simulink model "NGGenset_Test_System"  (R2013a)
settings: Solver=ode3  SolverMode=SingleTasking  StartTime=0.0  StopTime=150  FixedStep=Ts  RelTol=1e-3
PostLoadFcn:
  | Ts=50e-6;SIM_HIL=0;
InitFcn:
  | Ts=50e-6;SIM_HIL=0;
model workspace (MAT data in the model file):
  handle : class17 (value not decoded)
undefined symbols (not defined in the file): DiscIntNeverNeededParam, fdesignblkfcn, gcbh, Gen_900kW_external_control, Generator, HIL_GenSet, Left, NG_Genset_lib, ph, type, V
libraries: powerlib x33, simulink x30, powerlib_extras x24, rtio_opalrt_common x21, simulink_extras x6, dspsigops x6, breakers_1ph_3ph x6, rtio_generic_modbus x6, cables_lib x5, rteventslib x4, rtlab x2, ssn_lib x2
(part 3 of 4)

== system NGGenset_Test_System/SC_Console/Woodward/16TSDIn//16 TSDOut GR3/Din//Dout ch24-31 ==
  Bus Creator4 : BusCreator  Inputs=8
  times25 : Constant  Value=[0.05 0.15 0.25 0.35]
  times26 : Constant  Value=[0.1 0.2 0.3 0.4]
  times27 : Constant  Value=[0.15 0.25 0.35 0.45]
  times28 : Constant  Value=[0.2 0.3 0.4 0.5]
  times29 : Constant  Value=[0.25 0.35 0.45 0.55]
  times30 : Constant  Value=[0.3 0.4 0.5 0.6]
  times31 : Constant  Value=[0.3 0.4 0.5 0.6]
  times32 : Constant  Value=[0 0.1 0.2 0.3]
  Out1 : Outport
  wires:
  Bus Creator4/1 -> Out1/1
  times31/1 -> Bus Creator4/8  "times32"
  times30/1 -> Bus Creator4/7  "times31"
  times29/1 -> Bus Creator4/6  "times30"
  times28/1 -> Bus Creator4/5  "times29"
  times27/1 -> Bus Creator4/4  "times28"
  times26/1 -> Bus Creator4/3  "times27"
  times25/1 -> Bus Creator4/2  "times26"
  times32/1 -> Bus Creator4/1  "times25"

== system NGGenset_Test_System/SC_Console/Woodward/16TSDIn//16 TSDOut GR3/Dout state ctrl ==
  Bus Creator : BusCreator  Inputs=2
  Dout_CH16_CH23 : Subsystem
  Dout_CH24_CH31 : Subsystem
  Event State OUT : Outport
  wires:
  Dout_CH24_CH31/1(Dout_CH8_CH15) -> Bus Creator/2  "CH24-31"
  Dout_CH16_CH23/1(Dout_CH8_CH15) -> Bus Creator/1  "CH16-23"
  Bus Creator/1 -> Event State OUT/1

== system NGGenset_Test_System/SM_Master/Generator/NG Genset 3.5MVA/3.5MVA Generator with Primary Controllers1 ==
  wref : Inport
  Vtref : Inport  Port=2
  Enable : Inport  Port=3
  w_meas_Woodward : Inport  Port=4
  V_meas_Woodward : Inport  Port=5
  Woodward_Enable : Inport  Port=6
  Bus Creator1 : BusCreator
  Bus Creator3 : BusCreator  Inputs=3
  Bus Selector : BusSelector  OutputSignals=Vf_before,Vf_after
  NG Engine Speed & Voltage Control fast : Subsystem
  Synchronous Machine pu Fundamental : powerlib/Machines/Synchronous Machine pu Fundamental  PresetModel=No  MechanicalLoad=Mechanical power Pm  ShowDetailedParameters=on  RotorType=Salient-pole  NominalParameters=[3.5e+006 13800 60]  Stator=[0.008979 0.05 2.35 1.72]  Field=[0.00206 0.511]  Dampers2=[0.0652, 0.5134, 0.0287, 0.2553, 7.765e-3, 0.9167 ]  Dampers1=[0.2826 3.738 0.02545 0.2392]  Mechanical=[0.3468 0.009238 2]  PolePairs=2  InitialConditions="[ -99  0  0  0  0  0  0  0  0 ]"  SetSaturation=off  Saturation=[0.6404,0.7127,0.8441,0.9214,0.9956,1.082,1.19,1.316,1.457;0.7,0.7698,0.8872,0.9466,0.9969,1.046,1.1,1.151,1.201]  Units=per unit fundamental parameters  LoadFlowParameters=[1,0,0,0,0]  TsPowergui=0  TsBlock=-1  IterativeModel=Forward Euler  BusType=swing  Pref=0  Qref=0  Qmin=-inf  Qmax=inf  PLF=0  QLF=0
  A : PMIOPort  Port=1  Side=Right
  B : PMIOPort  Port=2  Side=Right
  C : PMIOPort  Port=3  Side=Right
  m : Outport
  Primary : Outport  Port=2
  Thermal data : Outport  Port=3
  wires:
  Woodward_Enable/1 -> NG Engine Speed & Voltage Control fast/7(Woodward Enable)
  Bus Creator3/1 -> Bus Creator1/2  "Vf"
  Bus Selector/2 -> Bus Creator3/3  "<Vf_after>"
  Bus Selector/1 -> Bus Creator3/2  "<Vf_before>"
  NG Engine Speed & Voltage Control fast/5(Misc) -> Bus Selector/1
  Bus Creator1/1 -> Primary/1
  NG Engine Speed & Voltage Control fast/4(w) -> Bus Creator1/4  "w"
  NG Engine Speed & Voltage Control fast/3(Vt) -> Bus Creator1/3  "vt"
  V_meas_Woodward/1 -> NG Engine Speed & Voltage Control fast/6(V_meas_Wood)
  w_meas_Woodward/1 -> NG Engine Speed & Voltage Control fast/5(w_meas_Wood)
  Synchronous Machine pu Fundamental/1 -> m/1, NG Engine Speed & Voltage Control fast/4(m)
  Enable/1 -> NG Engine Speed & Voltage Control fast/3(Generator Enable)
  NG Engine Speed & Voltage Control fast/1(Pm) -> Bus Creator1/1, Synchronous Machine pu Fundamental/1  "Pm"
  NG Engine Speed & Voltage Control fast/2(Vf) -> Bus Creator3/1, Synchronous Machine pu Fundamental/2  "vf"
  wref/1 -> NG Engine Speed & Voltage Control fast/1(wref)
  Vtref/1 -> NG Engine Speed & Voltage Control fast/2(Vtref)
  NG Engine Speed & Voltage Control fast/6(Themal data) -> Thermal data/1
  connections:
  Synchronous Machine pu Fundamental/RConn1 -- A/RConn1
  Synchronous Machine pu Fundamental/RConn2 -- B/RConn1
  Synchronous Machine pu Fundamental/RConn3 -- C/RConn1

== system NGGenset_Test_System/SM_Master/Generator/NG Genset 3.5MVA/Interface between Woodward Controller and simated generator ==
  note: Note: This may need a different scaling because it is the reference signal.
      | Reference has to be between 0.95 and 1.05 pu in order to be in tolerance.
  Woodward for wref : Inport
  Woodward for Vref : Inport  Port=2
  Add2 : Sum
  Add3 : Sum
  Gain2 : Gain
  Gain3 : Gain
  Mux1 : Mux  Inputs=2
  Vref_set : Constant  Value=0
  wref_set : Constant  Value=0
  wref,Vref : Outport
  wires:
  Gain2/1 -> Add2/1  "bias"
  Add2/1 -> Mux1/1
  Gain3/1 -> Add3/1  "bias"
  Vref_set/1 -> Add3/2
  Add3/1 -> Mux1/2
  Woodward for wref/1 -> Gain2/1
  Mux1/1 -> wref,Vref/1  "hardware"
  Woodward for Vref/1 -> Gain3/1
  wref_set/1 -> Add2/2

== system NGGenset_Test_System/SM_Master/Generator/NG Genset 3.5MVA/Simulated Generator Controller 3.5 MW ==
  Pref : Inport
  Qref : Inport  Port=2
  mode : Inport  Port=3
  set_vtref : Inport  Port=4
  set_wref : Inport  Port=5
  gen_m : Inport  Port=6
  Bus Selector1 : BusSelector  OutputSignals="Output active power   Peo (pu),Output reactive power  Qeo (pu)"
  Multiport Switch1 : MultiPortSwitch  DiagnosticForDefault=Warning
  Mux1 : Mux  Inputs=2
  Mux2 : Mux  Inputs=2
  Mux3 : Mux  Inputs=2
  PQ control : Subsystem
  PV control : Subsystem
  "wref, Vref" : Outport
  wires:
  Bus Selector1/1 -> PQ control/2(P (pu)), PV control/2(P (pu))  "<Output active power   Peo (pu)>"
  gen_m/1 -> Bus Selector1/1
  PQ control/1(w_ref (pu)) -> Mux1/1
  PQ control/2(V_ref (pu)) -> Mux1/2
  PV control/1(w_ref (pu)) -> Mux2/1
  set_vtref/1 -> Mux2/2, Mux3/2
  Mux1/1 -> Multiport Switch1/2
  Mux2/1 -> Multiport Switch1/3
  Mux3/1 -> Multiport Switch1/4
  Pref/1 -> PQ control/1(P_ref (pu)), PV control/1(P_ref (pu))
  Bus Selector1/2 -> PQ control/4(Q (pu))  "<Output reactive power  Qeo (pu)>"
  set_wref/1 -> Mux3/1
  Qref/1 -> PQ control/3(Q_ref (pu))
  mode/1 -> Multiport Switch1/1
  Multiport Switch1/1 -> "wref, Vref"/1

== system NGGenset_Test_System/SM_Master/Generator/NG Genset 3.5MVA/StabilityL ==
  Constant Load : powerlib/Elements/Three-Phase Parallel RLC Load  LConnTagsString=A|B|C  Configuration=Y (grounded)  NominalVoltage=v  NominalFrequency=60  ActivePower=kVA*1E3*pf  InductivePower=kVA*1E3*sqrt(1-pf^2)  CapacitivePower=0  Measurements=None  LoadType=constant Z
  A : PMIOPort  Port=1  Side=Left
  B : PMIOPort  Port=2  Side=Left
  C : PMIOPort  Port=3  Side=Left
  connections:
  A/RConn1 -- Constant Load/LConn1
  B/RConn1 -- Constant Load/LConn2
  C/RConn1 -- Constant Load/LConn3

== system NGGenset_Test_System/SM_Master/Generator/Woodward Inputs/Speed_System ==
  In1 : Inport
  Clock1 : Clock
      settings: DisableCoverage=on
  Duty : Constant  DisableCoverage=on  Value=0.5
  Gain1 : Gain  Gain=5
  Gain3 : Gain  Gain=5
  Gain4 : Gain  Gain=1800
  Output : Trigonometry
  Product1 : Product  DisableCoverage=on  SaturateOnIntegerOverflow=on  InputSameDT=on  OutDataTypeStr=Inherit: Same as first input
  Product3 : Product  DisableCoverage=on  SaturateOnIntegerOverflow=on  InputSameDT=on  OutDataTypeStr=Inherit: Same as first input
  RTE Conversion : rteventslib/Signal Attributes/RTE Conversion  inputdatatype=RTE Boolean  outputdatatype=Double  compensation=Disabled  nbMaxEvents=10  sampleTime=Ts
  RTE SPWM : rteventslib/Sources/RTE SPWM  NumberPhases=1-ph  CenterAlignmentMode=On  MaxFreq=inf  MinFreq=0  EnablingPort=off  ComplementaryMode=off  SpaceVector=off  RiseTimeDelay=0  MaxEvents=10  SampleTime=Ts
  initialFreq : Constant  DisableCoverage=on  Value=2*pi
  Out1 : Outport
  wires:
  Product1/1 -> Output/1
  Clock1/1 -> Product1/1
  initialFreq/1 -> Product3/1
  Product3/1 -> Product1/2
  Gain4/1 -> Product3/2, RTE SPWM/1
  Output/1 -> Gain3/1
  In1/1 -> Gain4/1
  RTE SPWM/1 -> RTE Conversion/1
  Duty/1 -> RTE SPWM/2
  RTE Conversion/1 -> Gain1/1
  Gain1/1 -> Out1/1

== system NGGenset_Test_System/SM_Master/Generator/Woodward Inputs/Speed_System1 ==
  In1 : Inport
  Clock1 : Clock
      settings: DisableCoverage=on
  Duty : Constant  DisableCoverage=on  Value=0.5
  Gain1 : Gain  Gain=5
  Gain3 : Gain  Gain=5
  Gain4 : Gain  Gain=1800
  Output : Trigonometry
  Product1 : Product  DisableCoverage=on  SaturateOnIntegerOverflow=on  InputSameDT=on  OutDataTypeStr=Inherit: Same as first input
  Product3 : Product  DisableCoverage=on  SaturateOnIntegerOverflow=on  InputSameDT=on  OutDataTypeStr=Inherit: Same as first input
  RTE Conversion : rteventslib/Signal Attributes/RTE Conversion  inputdatatype=RTE Boolean  outputdatatype=Double  compensation=Disabled  nbMaxEvents=10  sampleTime=Ts
  RTE SPWM : rteventslib/Sources/RTE SPWM  NumberPhases=1-ph  CenterAlignmentMode=On  MaxFreq=inf  MinFreq=0  EnablingPort=off  ComplementaryMode=off  SpaceVector=off  RiseTimeDelay=0  MaxEvents=10  SampleTime=Ts
  initialFreq : Constant  DisableCoverage=on  Value=2*pi
  Out1 : Outport
  wires:
  Product1/1 -> Output/1
  Clock1/1 -> Product1/1
  initialFreq/1 -> Product3/1
  Product3/1 -> Product1/2
  Gain4/1 -> Product3/2, RTE SPWM/1
  Output/1 -> Gain3/1
  In1/1 -> Gain4/1
  RTE SPWM/1 -> RTE Conversion/1
  Duty/1 -> RTE SPWM/2
  RTE Conversion/1 -> Gain1/1
  Gain1/1 -> Out1/1

== system NGGenset_Test_System/SM_Master/Generator/Woodward Outputs/DIO - Gr3 ==
  Dout : Inport
  Bus Creator : BusCreator  Inputs=2
  Bus Selector : BusSelector  OutputSignals=DI_CH00-07  OutputAsBus=on
  Bus Selector1 : BusSelector  OutputSignals=DI_CH08-15  OutputAsBus=on
  Conditioning : Subsystem
  Conditioning1 : Subsystem
  DigitalIn : rtio_opalrt_common/DigitalIn  CtrlName='OpCtrl'  portNb=5  FcnNos=Slot 3 Module A Subsection 1  size=1  maxcount=8  count=8  sampleTime=0  numchan=8
      settings: AttributesFormatString=%<CtrlName>
  DigitalIn1 : rtio_opalrt_common/DigitalIn  CtrlName='OpCtrl'  portNb=6  FcnNos=Slot 3 Module A Subsection 2  size=1  maxcount=8  count=8  sampleTime=0  numchan=8
      settings: AttributesFormatString=%<CtrlName>
  DigitalOut : rtio_opalrt_common/DigitalOut  CtrlName='OpCtrl'  portNb=5  FcnNos=Slot 3 Module B Subsection 1  size=1  maxcount=8  count=8  numchan=8
      settings: AttributesFormatString=%<CtrlName>
  DigitalOut1 : rtio_opalrt_common/DigitalOut  CtrlName='OpCtrl'  portNb=6  FcnNos=Slot 3 Module B Subsection 2  size=1  maxcount=8  count=8  numchan=8
      settings: AttributesFormatString=%<CtrlName>
  Terminator{1,3,5..6} (4 alike) : Terminator
  DIn : Outport
  wires:
  Conditioning1/1(Out1) -> Bus Creator/2
  Conditioning/1(Out1) -> Bus Creator/1
  Bus Creator/1 -> DIn/1
  DigitalIn1/1 -> Conditioning1/1(In1)  "DI_CH08-15"
  DigitalIn/1 -> Conditioning/1(In1)  "DI_CH00-07"
  DigitalIn1/2 -> Terminator6/1
  DigitalIn/2 -> Terminator5/1
  Bus Selector1/1 -> DigitalOut1/1
  Bus Selector/1 -> DigitalOut/1
  Dout/1 -> Bus Selector1/1, Bus Selector/1
  DigitalOut1/1 -> Terminator1/1
  DigitalOut/1 -> Terminator3/1

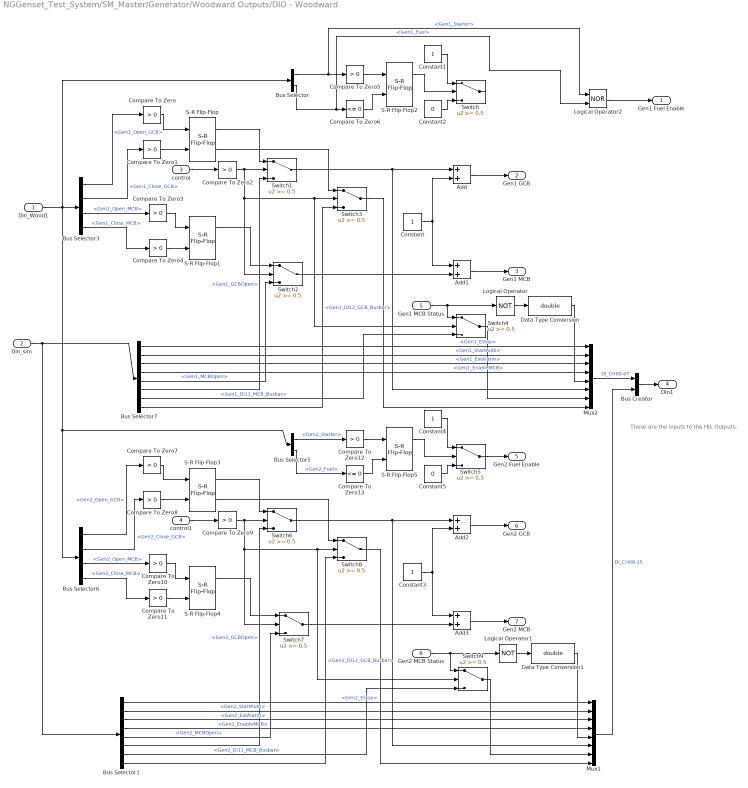
== system NGGenset_Test_System/SM_Master/Generator/Woodward Outputs/DIO - Woodward ==
  note: These are the inputs to
      | the HIL Outputs.
  Din_Wood1 : Inport
  Din_sim : Inport  Port=2
  control : Inport  Port=3
  control1 : Inport  Port=4
  Gen1 MCB Status : Inport  Port=5
  Gen2 MCB Status : Inport  Port=6
  Add{,1..3} (4 alike) : Sum
  Bus Creator : BusCreator  Inputs=2
  Bus Selector : BusSelector  OutputSignals=DI_CH00-07.Gen1_Starter,DI_CH00-07.Gen1_Fuel
  Bus Selector1 : BusSelector  OutputSignals=16 DOUT GR3.08-11.Gen2_Estop,16 DOUT GR3.08-11.Gen2_StartAuto,16 DOUT GR3.08-11.Gen2_ExtAlarm,16 DOUT GR3.08-11.Gen2_EnableMCB,16 DOUT GR3.12-15.Gen2_MCBOpen,16 DOUT GR3.12-15.Gen2_GCBOpen,16 DOUT GR3.12-15.Gen2_DI11_MCB_Busbar,16 DOUT GR3.12-15.Gen2_DI12_GCB_Busbar
  Bus Selector3 : BusSelector  OutputSignals=DI_CH00-07.Gen1_Open_GCB,DI_CH00-07.Gen1_Close_GCB,DI_CH00-07.Gen1_Open_MCB,DI_CH00-07.Gen1_Close_MCB
  Bus Selector5 : BusSelector  OutputSignals=DI_CH08-15.Gen2_Starter,DI_CH08-15.Gen2_Fuel
  Bus Selector6 : BusSelector  OutputSignals=DI_CH08-15.Gen2_Open_GCB,DI_CH08-15.Gen2_Close_GCB,DI_CH08-15.Gen2_Open_MCB,DI_CH08-15.Gen2_Close_MCB
  Bus Selector7 : BusSelector  OutputSignals=16 DOUT GR3.00-03.Gen1_Estop,16 DOUT GR3.00-03.Gen1_StartAuto,16 DOUT GR3.00-03.Gen1_ExtAlarm,16 DOUT GR3.00-03.Gen1_EnableMCB,16 DOUT GR3.04-07.Gen1_MCBOpen,16 DOUT GR3.04-07.Gen1_GCBOpen,16 DOUT GR3.04-07.Gen1_DI11_MCB_Busbar,16 DOUT GR3.04-07.Gen1_DI12_GCB_Busbar
  Compare To Zero{,1..5,7..12} (12 alike) : simulink/Logic and Bit Operations/Compare To Zero  relop=>  OutDataTypeStr=boolean
  Compare To Zero13 : simulink/Logic and Bit Operations/Compare To Zero  relop=<=  OutDataTypeStr=boolean
  Compare To Zero6 : simulink/Logic and Bit Operations/Compare To Zero  relop=<=  OutDataTypeStr=boolean
  Constant{,1,3..4} (4 alike) : Constant
  Constant2 : Constant  Value=0
  Constant5 : Constant  Value=0
  Data Type Conversion : DataTypeConversion  OutDataTypeStr=double
  Data Type Conversion1 : DataTypeConversion  OutDataTypeStr=double
  Logical Operator : Logic  Operator=NOT  AllPortsSameDT=off  OutDataTypeStr=boolean
  Logical Operator1 : Logic  Operator=NOT  AllPortsSameDT=off  OutDataTypeStr=boolean
  Logical Operator2 : Logic  Operator=NOR  AllPortsSameDT=off  OutDataTypeStr=boolean
  Mux1 : Mux  Inputs=8
  Mux2 : Mux  Inputs=8
  S-R Flip-Flop{,1,3..4} (4 alike) : simulink_extras/Flip Flops/S-R Flip-Flop  initial_condition=1
  S-R Flip-Flop2 : simulink_extras/Flip Flops/S-R Flip-Flop  initial_condition=0
  S-R Flip-Flop5 : simulink_extras/Flip Flops/S-R Flip-Flop  initial_condition=0
  Switch : Switch  Threshold=0.5
  Switch{1..4,6..9} (8 alike) : Switch  Threshold=0.5  OutDataTypeStr=double
      Switch8 settings: LockScale=on
  Switch5 : Switch  Threshold=0.5
  Gen1 Fuel Enable : Outport
  Gen1 GCB : Outport  Port=2
  Gen1 MCB : Outport  Port=3
  DIn1 : Outport  Port=4
  Gen2 Fuel Enable : Outport  Port=5
  Gen2 GCB : Outport  Port=6
  Gen2 MCB : Outport  Port=7
  wires:
  Logical Operator2/1 -> Gen1 Fuel Enable/1
  Data Type Conversion1/1 -> Mux1/5
  Logical Operator1/1 -> Data Type Conversion1/1
  Gen2 MCB Status/1 -> Switch9/1, Logical Operator1/1
  Logical Operator/1 -> Data Type Conversion/1
  Data Type Conversion/1 -> Mux2/5
  Gen1 MCB Status/1 -> Switch4/1, Logical Operator/1
  Switch8/1 -> Mux1/8
  Bus Selector1/8 -> Switch8/3  "<Gen2_DI12_GCB_Busbar>"
  Switch9/1 -> Mux1/7
  Bus Selector1/7 -> Switch9/3  "<Gen2_DI11_MCB_Busbar>"
  Switch3/1 -> Mux2/8
  Bus Selector7/8 -> Switch3/3  "<Gen1_DI12_GCB_Busbar>"
  Switch4/1 -> Mux2/7
  Bus Selector7/7 -> Switch4/3  "<Gen1_DI11_MCB_Busbar>"
  Din_sim/1 -> Bus Selector1/1, Bus Selector7/1
  Mux2/1 -> Bus Creator/1  "DI_CH00-07"
  Bus Selector7/6 -> Switch1/3  "<Gen1_GCBOpen>"
  Bus Selector7/5 -> Switch2/3  "<Gen1_MCBOpen>"
  Bus Selector7/4 -> Mux2/4  "<Gen1_EnableMCB>"
  Bus Selector7/3 -> Mux2/3  "<Gen1_ExtAlarm>"
  Bus Selector7/2 -> Mux2/2  "<Gen1_StartAuto>"
  Bus Selector7/1 -> Mux2/1  "<Gen1_Estop>"
  Bus Selector1/6 -> Switch6/3  "<Gen2_GCBOpen>"
  Bus Selector1/5 -> Switch7/3  "<Gen2_MCBOpen>"
  Bus Selector1/4 -> Mux1/4  "<Gen2_EnableMCB>"
  Bus Selector1/3 -> Mux1/3  "<Gen2_ExtAlarm>"
  Bus Selector1/2 -> Mux1/2  "<Gen2_StartAuto>"
  Bus Selector1/1 -> Mux1/1  "<Gen2_Estop>"
  Bus Selector3/3 -> Compare To Zero3/1  "<Gen1_Open_MCB>"
  Switch5/1 -> Gen2 Fuel Enable/1
  Compare To Zero13/1 -> S-R Flip-Flop5/2
  Constant4/1 -> Switch5/1
  Constant5/1 -> Switch5/3
  Compare To Zero12/1 -> S-R Flip-Flop5/1
  S-R Flip-Flop5/1 -> Switch5/2
  Bus Selector5/2 -> Compare To Zero13/1  "<Gen2_Fuel>"
  Bus Selector5/1 -> Compare To Zero12/1  "<Gen2_Starter>"
  Constant3/1 -> Add3/1, Add2/2
  Add3/1 -> Gen2 MCB/1
  Add2/1 -> Gen2 GCB/1
  S-R Flip-Flop3/2 -> Switch8/1
  Switch7/1 -> Add3/2
  Compare To Zero9/1 -> Switch9/2, Switch8/2, Switch7/2, Switch6/2
  Bus Selector6/2 -> Compare To Zero8/1  "<Gen2_Close_GCB>"
  S-R Flip-Flop4/1 -> Switch7/1
  Compare To Zero10/1 -> S-R Flip-Flop4/1
  Bus Selector6/3 -> Compare To Zero10/1  "<Gen2_Open_MCB>"
  Compare To Zero11/1 -> S-R Flip-Flop4/2
  Bus Selector6/4 -> Compare To Zero11/1  "<Gen2_Close_MCB>"
  Compare To Zero8/1 -> S-R Flip-Flop3/2
  Compare To Zero7/1 -> S-R Flip-Flop3/1
  Bus Selector6/1 -> Compare To Zero7/1  "<Gen2_Open_GCB>"
  Switch6/1 -> Mux1/6, Add2/1
  S-R Flip-Flop3/1 -> Switch6/1
  control1/1 -> Compare To Zero9/1
  Compare To Zero6/1 -> S-R Flip-Flop2/2
  Constant1/1 -> Switch/1
  Constant2/1 -> Switch/3
  Compare To Zero5/1 -> S-R Flip-Flop2/1
  S-R Flip-Flop2/1 -> Switch/2
  Bus Selector/2 -> Compare To Zero6/1, Logical Operator2/2  "<Gen1_Fuel>"
  Bus Selector/1 -> Compare To Zero5/1, Logical Operator2/1  "<Gen1_Starter>"
  Constant/1 -> Add1/1, Add/2
  Add1/1 -> Gen1 MCB/1
  Add/1 -> Gen1 GCB/1
  S-R Flip-Flop/2 -> Switch3/1
  Mux1/1 -> Bus Creator/2  "DI_CH08-15"
  Switch2/1 -> Add1/2
  Compare To Zero2/1 -> Switch4/2, Switch3/2, Switch2/2, Switch1/2
  S-R Flip-Flop1/1 -> Switch2/1
  Compare To Zero3/1 -> S-R Flip-Flop1/1
  Compare To Zero4/1 -> S-R Flip-Flop1/2
  Bus Selector3/4 -> Compare To Zero4/1  "<Gen1_Close_MCB>"
  Compare To Zero1/1 -> S-R Flip-Flop/2
  Compare To Zero/1 -> S-R Flip-Flop/1
  Switch1/1 -> Mux2/6, Add/1
  S-R Flip-Flop/1 -> Switch1/1
  Bus Creator/1 -> DIn1/1
  control/1 -> Compare To Zero2/1
  Din_Wood1/1 -> Bus Selector5/1, Bus Selector6/1, Bus Selector/1, Bus Selector3/1
  Bus Selector3/1 -> Compare To Zero/1  "<Gen1_Open_GCB>"
  Bus Selector3/2 -> Compare To Zero1/1  "<Gen1_Close_GCB>"

== system NGGenset_Test_System/SM_Master/Generator/Woodward Outputs/DOUT type config ==
  note: The Constants are used to select Digital Output type:
      | - 0: Time-Stamped Digital Output
      | - 1: Pulse-Width Modulated DIgital Output
  DataIn Send : rtio_opalrt_common/DataIn Send  CtrlName='OpCtrl'  FcnNos=11  width=1  portType=double  checkVersion=off  expectedId=0  expectedVersion=0  opComp=>=
      settings: AttributesFormatString=%<CtrlName>
  DataIn Send1 : rtio_opalrt_common/DataIn Send  CtrlName='OpCtrl'  FcnNos=12  width=1  portType=double  checkVersion=off  expectedId=0  expectedVersion=0  opComp=>=
      settings: AttributesFormatString=%<CtrlName>
  Subsection 3 DOUT type : Constant
  Subsection 4 DOUT type : Constant
  Terminator1 : Terminator
  Terminator2 : Terminator
  wires:
  DataIn Send/1 -> Terminator2/1
  DataIn Send1/1 -> Terminator1/1
  Subsection 4 DOUT type/1 -> DataIn Send1/1
  Subsection 3 DOUT type/1 -> DataIn Send/1

== system NGGenset_Test_System/SM_Master/Generator/Woodward Outputs/PWM IO - Gr3 ==
  PWMOut : Inport
  Bus Creator : BusCreator  Inputs=2
  Bus Creator1 : BusCreator  Inputs=2
  Bus Creator2 : BusCreator  Inputs=2
  Bus Selector : BusSelector  OutputSignals=FreqPWMOut16-23,DutyPWMOut16-23
  Bus Selector1 : BusSelector  OutputSignals=FreqPWMOut24-31,DutyPWMOut24-31
  Bus Selector2 : BusSelector  OutputSignals=16 PWMOUT GR3.Ch16-23,16 PWMOUT GR3.Ch24-31
  PWM In : rtio_opalrt_common/PWM In  CtrlName='OpCtrl'  portNb=9  FcnNos=Slot 3 Module A Subsection 3  maxCount=8  Count=8  sampleTime=0  numchan=8
      settings: AttributesFormatString=%<CtrlName>
  PWM In1 : rtio_opalrt_common/PWM In  CtrlName='OpCtrl'  portNb=10  FcnNos=Slot 3 Module A Subsection 4  maxCount=8  Count=8  sampleTime=0  numchan=8
      settings: AttributesFormatString=%<CtrlName>
  PWM Out : rtio_opalrt_common/PWM Out  CtrlName='OpCtrl'  portNb=9  FcnNos=Slot 3 Module B Subsection 3  size=64  maxcount=8  count=8  polarity=Active High  symMode=Symmetric  complementary=off  deadTime=0  numchan=8  loadnb=1  initphase=[0 0 0 0 0 0 0 0]
      settings: AttributesFormatString=%<CtrlName>
  PWM Out1 : rtio_opalrt_common/PWM Out  CtrlName='OpCtrl'  portNb=10  FcnNos=Slot 3 Module B Subsection 4  size=64  maxcount=8  count=8  polarity=Active High  symMode=Symmetric  complementary=off  deadTime=0  numchan=8  loadnb=2  initphase=[0 0 0 0 0 0 0 0]
      settings: AttributesFormatString=%<CtrlName>
  Terminator{,1,4..5} (4 alike) : Terminator
  PWMIn : Outport
  wires:
  Bus Selector2/2 -> Bus Selector1/1  "<Ch24-31>"
  PWM In1/2 -> Bus Creator2/2  "Duty"
  PWM In1/1 -> Bus Creator2/1  "Freq"
  PWM In/2 -> Bus Creator1/2  "Duty"
  PWM In/1 -> Bus Creator1/1  "Freq"
  PWM In/3 -> Terminator4/1
  PWM In1/3 -> Terminator5/1
  Bus Creator2/1 -> Bus Creator/2  "PWMI_CH24-31"
  Bus Creator1/1 -> Bus Creator/1  "PWMI_CH16-23"
  Bus Creator/1 -> PWMIn/1
  Bus Selector2/1 -> Bus Selector/1  "<Ch16-23>"
  PWMOut/1 -> Bus Selector2/1
  PWM Out1/1 -> Terminator1/1
  Bus Selector1/2 -> PWM Out1/2  "<DutyPWMOut24-31>"
  Bus Selector1/1 -> PWM Out1/1  "<FreqPWMOut24-31>"
  PWM Out/1 -> Terminator/1
  Bus Selector/2 -> PWM Out/2  "<DutyPWMOut16-23>"
  Bus Selector/1 -> PWM Out/1  "<FreqPWMOut16-23>"

== system NGGenset_Test_System/SM_Master/Generator/Woodward Outputs/TSDIO - Gr3 ==
  TSDout : Inport
  Bus Creator : BusCreator  Inputs=16
  Bus Creator1 : BusCreator  Inputs=16
  Bus Creator2 : BusCreator  Inputs=2
  Bus Selector : BusSelector  OutputSignals=16 TSDOUT GR3.states.CH16-23.states 17,16 TSDOUT GR3.times CH16-23.times17,16 TSDOUT GR3.states.CH16-23.states 18,16 TSDOUT GR3.times CH16-23.times18,16 TSDOUT GR3.states.CH16-23.states 19,16 TSDOUT GR3.times CH16-23.times19,16 TSDOUT GR3.states.CH16-23.states 20,16 TSDOUT GR3.times CH16-23.times20,16 TSDOUT GR3.states.CH16-23.states 21,16 TSDOUT GR3.times CH16-23.times21,16 TSDOUT GR3.states.CH16-23.states 22,16 TSDOUT GR3.times CH16-23.times22,16 TSDOUT GR3.states.CH16-23.states 23,16 TSDOUT GR3.times CH16-23.times23,16 TSDOUT GR3.states.CH16-23.states 24,16 TSDOUT GR3.times CH16-23.times24
  Bus Selector1 : BusSelector  OutputSignals=16 TSDOUT GR3.states.CH24-31.states 25,16 TSDOUT GR3.times CH24-31.times25,16 TSDOUT GR3.states.CH24-31.states 26,16 TSDOUT GR3.times CH24-31.times26,16 TSDOUT GR3.states.CH24-31.states 27,16 TSDOUT GR3.times CH24-31.times27,16 TSDOUT GR3.states.CH24-31.states 28,16 TSDOUT GR3.times CH24-31.times28,16 TSDOUT GR3.states.CH24-31.states 29,16 TSDOUT GR3.times CH24-31.times29,16 TSDOUT GR3.states.CH24-31.states 30,16 TSDOUT GR3.times CH24-31.times30,16 TSDOUT GR3.states.CH24-31.states 31,16 TSDOUT GR3.times CH24-31.times31,16 TSDOUT GR3.states.CH24-31.states 32,16 TSDOUT GR3.times CH24-31.times32
  EventDetector : rtio_opalrt_common/EventDetector  CtrlName='OpCtrl'  portNb=7  FcnNos=Slot 3 Module A Subsection 3  size=32  maxcount=8  nbChannels=8  width=4  timeUnit=Time ratio  sampleTime=0  numwidth=4
      settings: AttributesFormatString=%<CtrlName>
  EventDetector1 : rtio_opalrt_common/EventDetector  CtrlName='OpCtrl'  portNb=8  FcnNos=Slot 3 Module A Subsection 4  size=32  maxcount=8  nbChannels=8  width=4  timeUnit=Time ratio  sampleTime=0  numwidth=4
      settings: AttributesFormatString=%<CtrlName>
  EventGenerator : rtio_opalrt_common/EventGenerator  CtrlName='OpCtrl'  portNb=7  FcnNos=Slot 3 Module B Subsection 3  size=32  count=8  nbChannels=8  width=4  timeUnit=Time ratio  numwidth=4
      settings: AttributesFormatString=%<CtrlName>
  EventGenerator1 : rtio_opalrt_common/EventGenerator  CtrlName='OpCtrl'  portNb=8  FcnNos=Slot 3 Module B Subsection 4  size=32  count=8  nbChannels=8  width=4  timeUnit=Time ratio  numwidth=4
      settings: AttributesFormatString=%<CtrlName>
  Terminator{,1..3} (4 alike) : Terminator
  TSDin : Outport
  wires:
  Bus Creator2/1 -> TSDin/1  "TSDIN"
  Bus Creator/1 -> Bus Creator2/1  "CH16-23"
  EventDetector1/17 -> Terminator3/1  "states7"
  EventDetector1/1 -> Bus Creator1/1  "states1"
  EventDetector1/2 -> Bus Creator1/2  "times1"
  EventDetector1/3 -> Bus Creator1/3  "states2"
  EventDetector1/4 -> Bus Creator1/4  "times2"
  EventDetector1/5 -> Bus Creator1/5  "states1"
  EventDetector1/6 -> Bus Creator1/6  "times1"
  EventDetector1/7 -> Bus Creator1/7  "states2"
  EventDetector1/8 -> Bus Creator1/8  "times2"
  EventDetector1/9 -> Bus Creator1/9  "states3"
  EventDetector1/10 -> Bus Creator1/10  "times3"
  EventDetector1/11 -> Bus Creator1/11  "states4"
  EventDetector1/12 -> Bus Creator1/12  "times4"
  EventDetector1/13 -> Bus Creator1/13  "states5"
  EventDetector1/14 -> Bus Creator1/14  "times5"
  EventDetector1/15 -> Bus Creator1/15  "states6"
  EventDetector1/16 -> Bus Creator1/16  "times6"
  Bus Creator1/1 -> Bus Creator2/2  "CH24-31"
  Bus Selector1/16 -> EventGenerator1/16  "<times32>"
  Bus Selector1/15 -> EventGenerator1/15  "<states 32>"
  Bus Selector1/14 -> EventGenerator1/14  "<times31>"
  Bus Selector1/13 -> EventGenerator1/13  "<states 31>"
  Bus Selector1/12 -> EventGenerator1/12  "<times30>"
  Bus Selector1/11 -> EventGenerator1/11  "<states 30>"
  Bus Selector1/10 -> EventGenerator1/10  "<times29>"
  Bus Selector1/9 -> EventGenerator1/9  "<states 29>"
  Bus Selector1/8 -> EventGenerator1/8  "<times28>"
  Bus Selector1/7 -> EventGenerator1/7  "<states 28>"
  Bus Selector1/6 -> EventGenerator1/6  "<times27>"
  Bus Selector1/5 -> EventGenerator1/5  "<states 27>"
  Bus Selector1/4 -> EventGenerator1/4  "<times26>"
  Bus Selector1/3 -> EventGenerator1/3  "<states 26>"
  Bus Selector1/2 -> EventGenerator1/2  "<times25>"
  Bus Selector1/1 -> EventGenerator1/1  "<states 25>"
  EventGenerator1/1 -> Terminator2/1
  EventDetector/17 -> Terminator1/1
  EventDetector/1 -> Bus Creator/1  "states1"
  EventDetector/2 -> Bus Creator/2  "times1"
  EventDetector/3 -> Bus Creator/3  "states2"
  EventDetector/4 -> Bus Creator/4  "times2"
  EventDetector/5 -> Bus Creator/5  "states3"
  EventDetector/6 -> Bus Creator/6  "times3"
  EventDetector/7 -> Bus Creator/7  "states4"
  EventDetector/8 -> Bus Creator/8  "times4"
  EventDetector/9 -> Bus Creator/9  "states5"
  EventDetector/10 -> Bus Creator/10  "times5"
  EventDetector/11 -> Bus Creator/11  "states6"
  EventDetector/12 -> Bus Creator/12  "times6"
  EventDetector/13 -> Bus Creator/13  "states7"
  EventDetector/14 -> Bus Creator/14  "times7"
  EventDetector/15 -> Bus Creator/15  "states8"
  EventDetector/16 -> Bus Creator/16  "times8"
  EventGenerator/1 -> Terminator/1
  Bus Selector/1 -> EventGenerator/1  "<states 17>"
  Bus Selector/2 -> EventGenerator/2  "<times17>"
  Bus Selector/3 -> EventGenerator/3  "<states 18>"
  Bus Selector/4 -> EventGenerator/4  "<times18>"
  Bus Selector/5 -> EventGenerator/5  "<states 19>"
  Bus Selector/6 -> EventGenerator/6  "<times19>"
  Bus Selector/7 -> EventGenerator/7  "<states 20>"
  Bus Selector/8 -> EventGenerator/8  "<times20>"
  Bus Selector/9 -> EventGenerator/9  "<states 21>"
  Bus Selector/10 -> EventGenerator/10  "<times21>"
  Bus Selector/11 -> EventGenerator/11  "<states 22>"
  Bus Selector/12 -> EventGenerator/12  "<times22>"
  Bus Selector/13 -> EventGenerator/13  "<states 23>"
  Bus Selector/14 -> EventGenerator/14  "<times23>"
  Bus Selector/15 -> EventGenerator/15  "<states 24>"
  Bus Selector/16 -> EventGenerator/16  "<times24>"
  TSDout/1 -> Bus Selector1/1, Bus Selector/1

== system NGGenset_Test_System/SM_Master/Generator/Woodward Outputs/Woodward Primary Inputs ==
  Bias-ctrl : Inport
  Bus Creator : BusCreator
  Constant : Constant  Value=1.00
  Constant1 : Constant  Value=0
  Constant2 : Constant  Value=20
  Constant3 : Constant  Value=0
  Constant4 : Constant  Value=0
  Constant5 : Constant  Value=1.00
  Demux1 : Demux  Outputs=16
  Divide : Product  Inputs=*/
  Divide1 : Product  Inputs=*/
  GR1 B AIN (CH00-15) : Subsystem
  Lowpass Filter : Subsystem  DialogController=fdesignblkfcn  InitFcn=fdesignblkfcn(gcbh, {'InitFcn'});  mask(Lowpass Filter){}
      mask help: Design a lowpass filter
      settings: CopyFcn=fdesignblkfcn(gcbh, {'CopyFcn'});
      mask Help: helpview(mapfilelocation('dsp'), 'dsplowpassfilter');
      mask Display: disp('Lowpass')
  Lowpass Filter1 : Subsystem  DialogController=fdesignblkfcn  InitFcn=fdesignblkfcn(gcbh, {'InitFcn'});  mask(Lowpass Filter){}
      mask help: Design a lowpass filter
      settings: CopyFcn=fdesignblkfcn(gcbh, {'CopyFcn'});
      mask Help: helpview(mapfilelocation('dsp'), 'dsplowpassfilter');
      mask Display: disp('Lowpass')
  Sum : Sum  Inputs=|+-
  Sum1 : Sum  Inputs=|+-
  Switch : Switch  Threshold=0.5
  Switch1 : Switch  Threshold=0.5
  Gen1 Gov and AVR : Outport
  wires:
  Bus Creator/1 -> Gen1 Gov and AVR/1
  Constant/1 -> Bus Creator/1  "Gen1 Ref GOV"
  Constant5/1 -> Bus Creator/2  "Gen1 Ref AVR"
  Lowpass Filter1/1(Out) -> Switch1/1
  Lowpass Filter/1(Out) -> Switch/1
  Bias-ctrl/1 -> Switch1/2, Switch/2
  Constant1/1 -> Switch1/3, Switch/3
  Sum1/1 -> Lowpass Filter1/1(In)
  Switch1/1 -> Bus Creator/4  "Gen1 AVR"
  Switch/1 -> Bus Creator/3  "Gen1 Gov"
  Sum/1 -> Lowpass Filter/1(In)
  Constant4/1 -> Sum1/2
  Constant3/1 -> Sum/2
  Divide1/1 -> Sum1/1
  Divide/1 -> Sum/1
  Constant2/1 -> Divide/2, Divide1/2
  Demux1/2 -> Divide1/1
  Demux1/1 -> Divide/1
  GR1 B AIN (CH00-15)/1(Out1) -> Demux1/1, [AINs_Gr1]

== system NGGenset_Test_System/SM_Master/MODBUS1/SEL_787_Relay/PQ_Calculator ==
  Vabc : Inport
  Iabc : Inport  Port=2
  3-phase Instantaneous Active & Reactive Power : powerlib_extras/Measurements/3-phase  Instantaneous  Active & Reactive Power
  Demux : Demux  Outputs=2
  Discrete Mean value2 : powerlib_extras/Discrete Measurements/Discrete  Mean value  Freq=60  Vinit=0  Ts=Ts
  P : Outport
  Q : Outport  Port=2
  wires:
  3-phase Instantaneous Active & Reactive Power/1 -> Discrete Mean value2/1
  Discrete Mean value2/1 -> Demux/1
  Vabc/1 -> 3-phase Instantaneous Active & Reactive Power/1
  Iabc/1 -> 3-phase Instantaneous Active & Reactive Power/2
  Demux/1 -> P/1  "P"
  Demux/2 -> Q/1  "Q"

== system NGGenset_Test_System/SM_Master/MODBUS1/SEL_787_Relay/RMS_Calculator ==
  Signal : Inport
  Discrete Mean value6 : powerlib_extras/Discrete Measurements/Discrete  Mean value  Freq=60  Vinit=0  Ts=Ts
  Product3 : Product  RndMeth=Zero
  Signed Sqrt : Sqrt  SaturateOnIntegerOverflow=on
  RMS_Signal : Outport
  wires:
  Signal/1 -> Product3/1, Product3/2
  Product3/1 -> Discrete Mean value6/1
  Discrete Mean value6/1 -> Signed Sqrt/1
  Signed Sqrt/1 -> RMS_Signal/1

== system NGGenset_Test_System/SM_Master/MODBUS1/SEL_787_Relay/RMS_Calculator1 ==
  Signal : Inport
  Discrete Mean value6 : powerlib_extras/Discrete Measurements/Discrete  Mean value  Freq=60  Vinit=0  Ts=Ts
  Product3 : Product  RndMeth=Zero
  Signed Sqrt : Sqrt  SaturateOnIntegerOverflow=on
  RMS_Signal : Outport
  wires:
  Signal/1 -> Product3/1, Product3/2
  Product3/1 -> Discrete Mean value6/1
  Discrete Mean value6/1 -> Signed Sqrt/1
  Signed Sqrt/1 -> RMS_Signal/1

== system NGGenset_Test_System/SM_Master/MODBUS1/SEL_787_Relay/pf_Calculator ==
  P : Inport
  Q : Inport  Port=2
  Fcn : Fcn  Expr=u(1) / sqrt(u(1)^2 + u(2)^2)
  Fcn1 : Fcn  Expr=sqrt(u(1)^2 + u(2)^2)
  Mux : Mux  Inputs=2
  Mux1 : Mux  Inputs=2
  Scope : Scope
      settings: YMin=0.8475  YMax=0.875  SaveName=ScopeData2
  pf : Outport
  S : Outport  Port=2
  wires:
  Fcn1/1 -> S/1
  Mux1/1 -> Fcn1/1
  Fcn/1 -> Scope/1, pf/1
  Mux/1 -> Fcn/1
  P/1 -> Mux1/1, Mux/1
  Q/1 -> Mux1/2, Mux/2

== system NGGenset_Test_System/SM_Master/MODBUS2/SEL_787_Relay/PQ_Calculator ==
  Vabc : Inport
  Iabc : Inport  Port=2
  3-phase Instantaneous Active & Reactive Power : powerlib_extras/Measurements/3-phase  Instantaneous  Active & Reactive Power
  Demux : Demux  Outputs=2
  Discrete Mean value2 : powerlib_extras/Discrete Measurements/Discrete  Mean value  Freq=60  Vinit=0  Ts=Ts
  P : Outport
  Q : Outport  Port=2
  wires:
  3-phase Instantaneous Active & Reactive Power/1 -> Discrete Mean value2/1
  Discrete Mean value2/1 -> Demux/1
  Vabc/1 -> 3-phase Instantaneous Active & Reactive Power/1
  Iabc/1 -> 3-phase Instantaneous Active & Reactive Power/2
  Demux/1 -> P/1  "P"
  Demux/2 -> Q/1  "Q"

== system NGGenset_Test_System/SM_Master/MODBUS2/SEL_787_Relay/RMS_Calculator ==
  Signal : Inport
  Discrete Mean value6 : powerlib_extras/Discrete Measurements/Discrete  Mean value  Freq=60  Vinit=0  Ts=Ts
  Product3 : Product  RndMeth=Zero
  Signed Sqrt : Sqrt  SaturateOnIntegerOverflow=on
  RMS_Signal : Outport
  wires:
  Signal/1 -> Product3/1, Product3/2
  Product3/1 -> Discrete Mean value6/1
  Discrete Mean value6/1 -> Signed Sqrt/1
  Signed Sqrt/1 -> RMS_Signal/1

== system NGGenset_Test_System/SM_Master/MODBUS2/SEL_787_Relay/RMS_Calculator1 ==
  Signal : Inport
  Discrete Mean value6 : powerlib_extras/Discrete Measurements/Discrete  Mean value  Freq=60  Vinit=0  Ts=Ts
  Product3 : Product  RndMeth=Zero
  Signed Sqrt : Sqrt  SaturateOnIntegerOverflow=on
  RMS_Signal : Outport
  wires:
  Signal/1 -> Product3/1, Product3/2
  Product3/1 -> Discrete Mean value6/1
  Discrete Mean value6/1 -> Signed Sqrt/1
  Signed Sqrt/1 -> RMS_Signal/1

== system NGGenset_Test_System/SM_Master/MODBUS2/SEL_787_Relay/pf_Calculator ==
  P : Inport
  Q : Inport  Port=2
  Fcn : Fcn  Expr=u(1) / sqrt(u(1)^2 + u(2)^2)
  Fcn1 : Fcn  Expr=sqrt(u(1)^2 + u(2)^2)
  Mux : Mux  Inputs=2
  Mux1 : Mux  Inputs=2
  Scope : Scope
      settings: YMin=0.8475  YMax=0.875  SaveName=ScopeData2
  pf : Outport
  S : Outport  Port=2
  wires:
  Fcn1/1 -> S/1
  Mux1/1 -> Fcn1/1
  Fcn/1 -> Scope/1, pf/1
  Mux/1 -> Fcn/1
  P/1 -> Mux1/1, Mux/1
  Q/1 -> Mux1/2, Mux/2

== system NGGenset_Test_System/SM_Master/MODBUS4/SEL_787_Relay/PQ_Calculator ==
  Vabc : Inport
  Iabc : Inport  Port=2
  3-phase Instantaneous Active & Reactive Power : powerlib_extras/Measurements/3-phase  Instantaneous  Active & Reactive Power
  Demux : Demux  Outputs=2
  Discrete Mean value2 : powerlib_extras/Discrete Measurements/Discrete  Mean value  Freq=60  Vinit=0  Ts=Ts
  P : Outport
  Q : Outport  Port=2
  wires:
  3-phase Instantaneous Active & Reactive Power/1 -> Discrete Mean value2/1
  Discrete Mean value2/1 -> Demux/1
  Vabc/1 -> 3-phase Instantaneous Active & Reactive Power/1
  Iabc/1 -> 3-phase Instantaneous Active & Reactive Power/2
  Demux/1 -> P/1  "P"
  Demux/2 -> Q/1  "Q"

== system NGGenset_Test_System/SM_Master/MODBUS4/SEL_787_Relay/RMS_Calculator ==
  Signal : Inport
  Discrete Mean value6 : powerlib_extras/Discrete Measurements/Discrete  Mean value  Freq=60  Vinit=0  Ts=Ts
  Product3 : Product  RndMeth=Zero
  Signed Sqrt : Sqrt  SaturateOnIntegerOverflow=on
  RMS_Signal : Outport
  wires:
  Signal/1 -> Product3/1, Product3/2
  Product3/1 -> Discrete Mean value6/1
  Discrete Mean value6/1 -> Signed Sqrt/1
  Signed Sqrt/1 -> RMS_Signal/1

== system NGGenset_Test_System/SM_Master/MODBUS4/SEL_787_Relay/RMS_Calculator1 ==
  Signal : Inport
  Discrete Mean value6 : powerlib_extras/Discrete Measurements/Discrete  Mean value  Freq=60  Vinit=0  Ts=Ts
  Product3 : Product  RndMeth=Zero
  Signed Sqrt : Sqrt  SaturateOnIntegerOverflow=on
  RMS_Signal : Outport
  wires:
  Signal/1 -> Product3/1, Product3/2
  Product3/1 -> Discrete Mean value6/1
  Discrete Mean value6/1 -> Signed Sqrt/1
  Signed Sqrt/1 -> RMS_Signal/1

== system NGGenset_Test_System/SM_Master/MODBUS4/SEL_787_Relay/pf_Calculator ==
  P : Inport
  Q : Inport  Port=2
  Fcn : Fcn  Expr=u(1) / sqrt(u(1)^2 + u(2)^2)
  Fcn1 : Fcn  Expr=sqrt(u(1)^2 + u(2)^2)
  Mux : Mux  Inputs=2
  Mux1 : Mux  Inputs=2
  Scope : Scope
      settings: YMin=0.8475  YMax=0.875  SaveName=ScopeData2
  pf : Outport
  S : Outport  Port=2
  wires:
  Fcn1/1 -> S/1
  Mux1/1 -> Fcn1/1
  Fcn/1 -> Scope/1, pf/1
  Mux/1 -> Fcn/1
  P/1 -> Mux1/1, Mux/1
  Q/1 -> Mux1/2, Mux/2

== system NGGenset_Test_System/SM_Master/MODBUS5/SEL_787_Relay/PQ_Calculator ==
  Vabc : Inport
  Iabc : Inport  Port=2
  3-phase Instantaneous Active & Reactive Power : powerlib_extras/Measurements/3-phase  Instantaneous  Active & Reactive Power
  Demux : Demux  Outputs=2
  Discrete Mean value2 : powerlib_extras/Discrete Measurements/Discrete  Mean value  Freq=60  Vinit=0  Ts=Ts
  P : Outport
  Q : Outport  Port=2
  wires:
  3-phase Instantaneous Active & Reactive Power/1 -> Discrete Mean value2/1
  Discrete Mean value2/1 -> Demux/1
  Vabc/1 -> 3-phase Instantaneous Active & Reactive Power/1
  Iabc/1 -> 3-phase Instantaneous Active & Reactive Power/2
  Demux/1 -> P/1  "P"
  Demux/2 -> Q/1  "Q"

== system NGGenset_Test_System/SM_Master/MODBUS5/SEL_787_Relay/RMS_Calculator ==
  Signal : Inport
  Discrete Mean value6 : powerlib_extras/Discrete Measurements/Discrete  Mean value  Freq=60  Vinit=0  Ts=Ts
  Product3 : Product  RndMeth=Zero
  Signed Sqrt : Sqrt  SaturateOnIntegerOverflow=on
  RMS_Signal : Outport
  wires:
  Signal/1 -> Product3/1, Product3/2
  Product3/1 -> Discrete Mean value6/1
  Discrete Mean value6/1 -> Signed Sqrt/1
  Signed Sqrt/1 -> RMS_Signal/1

== system NGGenset_Test_System/SM_Master/MODBUS5/SEL_787_Relay/RMS_Calculator1 ==
  Signal : Inport
  Discrete Mean value6 : powerlib_extras/Discrete Measurements/Discrete  Mean value  Freq=60  Vinit=0  Ts=Ts
  Product3 : Product  RndMeth=Zero
  Signed Sqrt : Sqrt  SaturateOnIntegerOverflow=on
  RMS_Signal : Outport
  wires:
  Signal/1 -> Product3/1, Product3/2
  Product3/1 -> Discrete Mean value6/1
  Discrete Mean value6/1 -> Signed Sqrt/1
  Signed Sqrt/1 -> RMS_Signal/1

== system NGGenset_Test_System/SM_Master/MODBUS5/SEL_787_Relay/pf_Calculator ==
  P : Inport
  Q : Inport  Port=2
  Fcn : Fcn  Expr=u(1) / sqrt(u(1)^2 + u(2)^2)
  Fcn1 : Fcn  Expr=sqrt(u(1)^2 + u(2)^2)
  Mux : Mux  Inputs=2
  Mux1 : Mux  Inputs=2
  Scope : Scope
      settings: YMin=0.8475  YMax=0.875  SaveName=ScopeData2
  pf : Outport
  S : Outport  Port=2
  wires:
  Fcn1/1 -> S/1
  Mux1/1 -> Fcn1/1
  Fcn/1 -> Scope/1, pf/1
  Mux/1 -> Fcn/1
  P/1 -> Mux1/1, Mux/1
  Q/1 -> Mux1/2, Mux/2

== system NGGenset_Test_System/SM_Master/MODBUS6/SEL_787_Relay/PQ_Calculator ==
  Vabc : Inport
  Iabc : Inport  Port=2
  3-phase Instantaneous Active & Reactive Power : powerlib_extras/Measurements/3-phase  Instantaneous  Active & Reactive Power
  Demux : Demux  Outputs=2
  Discrete Mean value2 : powerlib_extras/Discrete Measurements/Discrete  Mean value  Freq=60  Vinit=0  Ts=Ts
  P : Outport
  Q : Outport  Port=2
  wires:
  3-phase Instantaneous Active & Reactive Power/1 -> Discrete Mean value2/1
  Discrete Mean value2/1 -> Demux/1
  Vabc/1 -> 3-phase Instantaneous Active & Reactive Power/1
  Iabc/1 -> 3-phase Instantaneous Active & Reactive Power/2
  Demux/1 -> P/1  "P"
  Demux/2 -> Q/1  "Q"

== system NGGenset_Test_System/SM_Master/MODBUS6/SEL_787_Relay/RMS_Calculator ==
  Signal : Inport
  Discrete Mean value6 : powerlib_extras/Discrete Measurements/Discrete  Mean value  Freq=60  Vinit=0  Ts=Ts
  Product3 : Product  RndMeth=Zero
  Signed Sqrt : Sqrt  SaturateOnIntegerOverflow=on
  RMS_Signal : Outport
  wires:
  Signal/1 -> Product3/1, Product3/2
  Product3/1 -> Discrete Mean value6/1
  Discrete Mean value6/1 -> Signed Sqrt/1
  Signed Sqrt/1 -> RMS_Signal/1

== system NGGenset_Test_System/SM_Master/MODBUS6/SEL_787_Relay/RMS_Calculator1 ==
  Signal : Inport
  Discrete Mean value6 : powerlib_extras/Discrete Measurements/Discrete  Mean value  Freq=60  Vinit=0  Ts=Ts
  Product3 : Product  RndMeth=Zero
  Signed Sqrt : Sqrt  SaturateOnIntegerOverflow=on
  RMS_Signal : Outport
  wires:
  Signal/1 -> Product3/1, Product3/2
  Product3/1 -> Discrete Mean value6/1
  Discrete Mean value6/1 -> Signed Sqrt/1
  Signed Sqrt/1 -> RMS_Signal/1

== system NGGenset_Test_System/SM_Master/MODBUS6/SEL_787_Relay/pf_Calculator ==
  P : Inport
  Q : Inport  Port=2
  Fcn : Fcn  Expr=u(1) / sqrt(u(1)^2 + u(2)^2)
  Fcn1 : Fcn  Expr=sqrt(u(1)^2 + u(2)^2)
  Mux : Mux  Inputs=2
  Mux1 : Mux  Inputs=2
  Scope : Scope
      settings: YMin=0.8475  YMax=0.875  SaveName=ScopeData2
  pf : Outport
  S : Outport  Port=2
  wires:
  Fcn1/1 -> S/1
  Mux1/1 -> Fcn1/1
  Fcn/1 -> Scope/1, pf/1
  Mux/1 -> Fcn/1
  P/1 -> Mux1/1, Mux/1
  Q/1 -> Mux1/2, Mux/2

== system NGGenset_Test_System/SM_Master/MODBUS8/SEL_787_Relay/PQ_Calculator ==
  Vabc : Inport
  Iabc : Inport  Port=2
  3-phase Instantaneous Active & Reactive Power : powerlib_extras/Measurements/3-phase  Instantaneous  Active & Reactive Power
  Demux : Demux  Outputs=2
  Discrete Mean value2 : powerlib_extras/Discrete Measurements/Discrete  Mean value  Freq=60  Vinit=0  Ts=Ts
  P : Outport
  Q : Outport  Port=2
  wires:
  3-phase Instantaneous Active & Reactive Power/1 -> Discrete Mean value2/1
  Discrete Mean value2/1 -> Demux/1
  Vabc/1 -> 3-phase Instantaneous Active & Reactive Power/1
  Iabc/1 -> 3-phase Instantaneous Active & Reactive Power/2
  Demux/1 -> P/1  "P"
  Demux/2 -> Q/1  "Q"

== system NGGenset_Test_System/SM_Master/MODBUS8/SEL_787_Relay/RMS_Calculator ==
  Signal : Inport
  Discrete Mean value6 : powerlib_extras/Discrete Measurements/Discrete  Mean value  Freq=60  Vinit=0  Ts=Ts
  Product3 : Product  RndMeth=Zero
  Signed Sqrt : Sqrt  SaturateOnIntegerOverflow=on
  RMS_Signal : Outport
  wires:
  Signal/1 -> Product3/1, Product3/2
  Product3/1 -> Discrete Mean value6/1
  Discrete Mean value6/1 -> Signed Sqrt/1
  Signed Sqrt/1 -> RMS_Signal/1

== system NGGenset_Test_System/SM_Master/MODBUS8/SEL_787_Relay/RMS_Calculator1 ==
  Signal : Inport
  Discrete Mean value6 : powerlib_extras/Discrete Measurements/Discrete  Mean value  Freq=60  Vinit=0  Ts=Ts
  Product3 : Product  RndMeth=Zero
  Signed Sqrt : Sqrt  SaturateOnIntegerOverflow=on
  RMS_Signal : Outport
  wires:
  Signal/1 -> Product3/1, Product3/2
  Product3/1 -> Discrete Mean value6/1
  Discrete Mean value6/1 -> Signed Sqrt/1
  Signed Sqrt/1 -> RMS_Signal/1

== system NGGenset_Test_System/SM_Master/MODBUS8/SEL_787_Relay/pf_Calculator ==
  P : Inport
  Q : Inport  Port=2
  Fcn : Fcn  Expr=u(1) / sqrt(u(1)^2 + u(2)^2)
  Fcn1 : Fcn  Expr=sqrt(u(1)^2 + u(2)^2)
  Mux : Mux  Inputs=2
  Mux1 : Mux  Inputs=2
  Scope : Scope
      settings: YMin=0.8475  YMax=0.875  SaveName=ScopeData2
  pf : Outport
  S : Outport  Port=2
  wires:
  Fcn1/1 -> S/1
  Mux1/1 -> Fcn1/1
  Fcn/1 -> Scope/1, pf/1
  Mux/1 -> Fcn/1
  P/1 -> Mux1/1, Mux/1
  Q/1 -> Mux1/2, Mux/2

== system NGGenset_Test_System/SC_Console/Woodward/16TSDIn//16 TSDOut GR3/Dout state ctrl/Dout_CH16_CH23 ==
  Bus Creator1 : BusCreator  Inputs=8
  Dout_CH{16..23} (8 alike) : Constant  Value=[1 0 1 0]
  Manual Switch{17..24} (8 alike) : ManualSwitch
  Zero_Dout_CH{16..23} (8 alike) : Constant  Value=[0 0 0 0]
  Dout_CH8_CH15 : Outport
  wires:
  Manual Switch24/1 -> Bus Creator1/8  "states 24"
  Manual Switch23/1 -> Bus Creator1/7  "states 23"
  Manual Switch22/1 -> Bus Creator1/6  "states 22"
  Manual Switch21/1 -> Bus Creator1/5  "states 21"
  Manual Switch20/1 -> Bus Creator1/4  "states 20"
  Manual Switch19/1 -> Bus Creator1/3  "states 19"
  Manual Switch18/1 -> Bus Creator1/2  "states 18"
  Manual Switch17/1 -> Bus Creator1/1  "states 17"
  Zero_Dout_CH23/1 -> Manual Switch24/2
  Dout_CH23/1 -> Manual Switch24/1
  Zero_Dout_CH22/1 -> Manual Switch23/2
  Dout_CH22/1 -> Manual Switch23/1
  Zero_Dout_CH21/1 -> Manual Switch22/2
  Dout_CH21/1 -> Manual Switch22/1
  Zero_Dout_CH20/1 -> Manual Switch21/2
  Dout_CH20/1 -> Manual Switch21/1
  Zero_Dout_CH19/1 -> Manual Switch20/2
  Dout_CH19/1 -> Manual Switch20/1
  Zero_Dout_CH18/1 -> Manual Switch19/2
  Dout_CH18/1 -> Manual Switch19/1
  Zero_Dout_CH17/1 -> Manual Switch18/2
  Dout_CH17/1 -> Manual Switch18/1
  Zero_Dout_CH16/1 -> Manual Switch17/2
  Dout_CH16/1 -> Manual Switch17/1
  Bus Creator1/1 -> Dout_CH8_CH15/1

== system NGGenset_Test_System/SC_Console/Woodward/16TSDIn//16 TSDOut GR3/Dout state ctrl/Dout_CH24_CH31 ==
  Bus Creator : BusCreator  Inputs=8
  Dout_CH{24..31} (8 alike) : Constant  Value=[1 0 1 0]
  Manual Switch{25..32} (8 alike) : ManualSwitch
  Zero_Dout_CH{24..31} (8 alike) : Constant  Value=[0 0 0 0]
  Dout_CH8_CH15 : Outport
  wires:
  Bus Creator/1 -> Dout_CH8_CH15/1
  Dout_CH24/1 -> Manual Switch25/1
  Zero_Dout_CH24/1 -> Manual Switch25/2
  Dout_CH25/1 -> Manual Switch26/1
  Zero_Dout_CH25/1 -> Manual Switch26/2
  Dout_CH26/1 -> Manual Switch27/1
  Zero_Dout_CH26/1 -> Manual Switch27/2
  Dout_CH27/1 -> Manual Switch28/1
  Zero_Dout_CH27/1 -> Manual Switch28/2
  Dout_CH28/1 -> Manual Switch29/1
  Zero_Dout_CH28/1 -> Manual Switch29/2
  Dout_CH29/1 -> Manual Switch30/1
  Zero_Dout_CH29/1 -> Manual Switch30/2
  Dout_CH30/1 -> Manual Switch31/1
  Zero_Dout_CH30/1 -> Manual Switch31/2
  Dout_CH31/1 -> Manual Switch32/1
  Zero_Dout_CH31/1 -> Manual Switch32/2
  Manual Switch25/1 -> Bus Creator/1  "states 25"
  Manual Switch26/1 -> Bus Creator/2  "states 26"
  Manual Switch27/1 -> Bus Creator/3  "states 27"
  Manual Switch28/1 -> Bus Creator/4  "states 28"
  Manual Switch29/1 -> Bus Creator/5  "states 29"
  Manual Switch30/1 -> Bus Creator/6  "states 30"
  Manual Switch31/1 -> Bus Creator/7  "states 31"
  Manual Switch32/1 -> Bus Creator/8  "states 32"
